simulink model "cruise_ctrl_RL"  (R2021a)
settings: Solver=FixedStepAuto  StartTime=0.0  StopTime=Tf  FixedStep=0.1  RelTol=1e-3
values from neighbouring files (symbols this model uses):
  A = 2.4    [init_cc.m]
  alpha = [40, 25, 16, 12, 10]    [init_cc.m]    (also in main_script_random.m = 0.5)
  beta = 0.4    [init_cc.m]
  Cd = 0.32    [init_cc.m]
  Cr = 0.01    [init_cc.m]
  g = 9.8    [init_cc.m]
  gear = 4    [init_cc.m]
  m = 1000    [init_cc.m]
  rho = 1.3    [init_cc.m]
  Tm = 190    [init_cc.m]
  Ts = 1    [model_myscript.m]    (also in model_myscript_3layer.m)
  wm = 420    [init_cc.m]
undefined symbols (not defined in the file or in its folder): DiscIntNeverNeededParam, phi_cc
libraries: simulink x3, rllib x1
settings Model: Creator=nikhil  LastModifiedBy=nikhil
settings SolverCC: AlgebraicLoopSolver=TrustRegion
settings DataIOCC: ReturnWorkspaceOutputs=off
settings DebuggingCC: SFMachineParentedDataDiag=warning  ArithmeticOperatorsInVariantConditions=warning
settings SFSimCC: SimUseLocalCustomCode=off  CustomCodeUndefinedFunction=UseInterfaceOnly
settings RTWCC: RTWUseLocalCustomCode=off
settings CodeAppCC: StateflowObjectComments=on

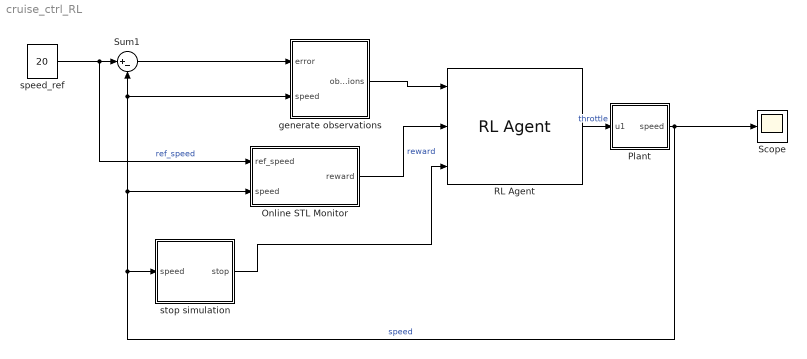
== system cruise_ctrl_RL ==
  Online STL Monitor : Subsystem
  Plant : Subsystem
  RL Agent : rllib/RL Agent  Agent=agent  ExternalActionAsInput=off  ProvideCumRwd=off  TreatAsDirectFeedthrough=on
  Scope : Scope
  Sum1 : Sum  Inputs=|+-  SaturateOnIntegerOverflow=on
  generate observations : Subsystem
  speed_ref : Constant  Value=20
  stop simulation : Subsystem
  wires:
  Plant/1(speed) -> Scope/1, stop simulation/1(speed), Online STL Monitor/2(speed), generate observations/2(speed), Sum1/2  "speed"
  RL Agent/1 -> Plant/1(u1)  "throttle"
  speed_ref/1 -> Online STL Monitor/1(ref_speed), Sum1/1  "ref_speed"
  stop simulation/1(stop) -> RL Agent/3
  generate observations/1(observations) -> RL Agent/1
  Sum1/1 -> generate observations/1(error)
  Online STL Monitor/1(reward) -> RL Agent/2  "reward"

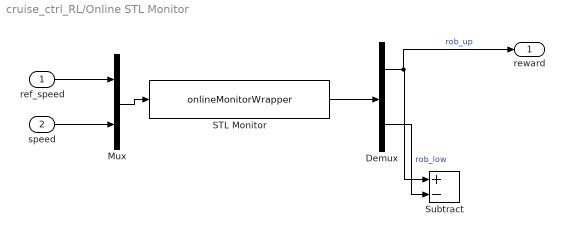
== system cruise_ctrl_RL/Online STL Monitor ==
  ref_speed : Inport
  speed : Inport  Port=2
  Demux : Demux  Outputs=2
  Mux : Mux  Inputs=2
  STL Monitor : S-Function  FunctionName=onlineMonitorWrapper  Parameters=SignalNames, STLString, MaxRob,RefreshRate  SFunctionDeploymentMode=off  EnableBusSupport=off  mask(STL Monitor){SignalNames='ref_speed,speed', STLString=phi_cc, MaxRob=100, RefreshRate=0.1}
      mask prompts: SignalNames "Signal names"; STLString "String For STL formula"; MaxRob "Maximum robustness"; RefreshRate "Refresh Rate"
      mask help:
      | Monitor an STL Formula on input signal. Takes two parameters: a string with
      | comma separated identifiers for the input signals, (ex: 'x1,x2,y'), and a
      | string for the formula (ex: 'alw_[0, 50] (x1[t]>0 => y[t] >0)'). Outputs a
      | two dimensional signal bounding the satisfaction of the formula.
      mask Display: fprintf('%s', STLString)
  Subtract : Sum  Inputs=+-
  reward : Outport
  wires:
  Mux/1 -> STL Monitor/1
  STL Monitor/1 -> Demux/1
  Demux/2 -> Subtract/2  "rob_low"
  Demux/1 -> reward/1, Subtract/1  "rob_up"
  speed/1 -> Mux/2
  ref_speed/1 -> Mux/1

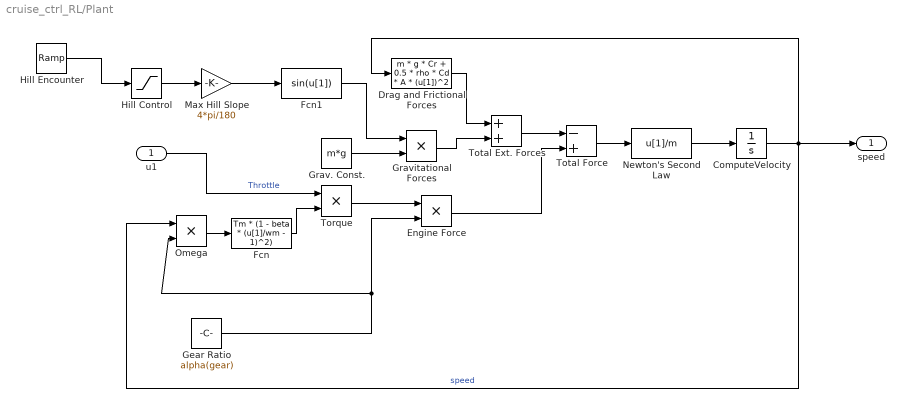
== system cruise_ctrl_RL/Plant ==
  u1 : Inport
  ComputeVelocity : Integrator  InitialCondition=10
  Drag and Frictional Forces : Fcn  Expr=m * g * Cr + 0.5 * rho * Cd * A * (u[1])^2
  Engine Force : Product  Inputs=**
  Fcn : Fcn  Expr=Tm * (1 - beta * (u[1]/wm - 1)^2)
  Fcn1 : Fcn
  Gear Ratio : Constant  Value=alpha(gear)
  Grav. Const. : Constant  Value=m*g
  Gravitational Forces : Product  RndMeth=Zero
  Hill Control : Saturate  UpperLimit=1  LowerLimit=0
  Hill Encounter : simulink/Sources/Ramp  slope=1  start=60  InitialOutput=0
  Max Hill Slope : Gain  Gain=4*pi/180
  Newton's Second Law : Fcn  Expr=u[1]/m
  Omega : Product  RndMeth=Zero
  Torque : Product  RndMeth=Zero
  Total Ext. Forces : Sum
  Total Force : Sum  Inputs=-+
  speed : Outport
  wires:
  Max Hill Slope/1 -> Fcn1/1
  Engine Force/1 -> Total Force/2
  Total Force/1 -> Newton's Second Law/1
  Gravitational Forces/1 -> Total Ext. Forces/2
  Gear Ratio/1 -> Engine Force/2, Omega/2
  Drag and Frictional Forces/1 -> Total Ext. Forces/1
  Total Ext. Forces/1 -> Total Force/1
  Fcn/1 -> Torque/2
  Hill Control/1 -> Max Hill Slope/1
  Hill Encounter/1 -> Hill Control/1
  Fcn1/1 -> Gravitational Forces/1
  Grav. Const./1 -> Gravitational Forces/2
  u1/1 -> Torque/1  "Throttle"
  Torque/1 -> Engine Force/1
  Newton's Second Law/1 -> ComputeVelocity/1
  Omega/1 -> Fcn/1
  ComputeVelocity/1 -> speed/1, Drag and Frictional Forces/1, Omega/1  "speed"

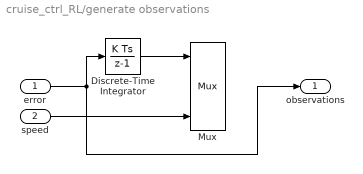
== system cruise_ctrl_RL/generate observations ==
  error : Inport
  speed : Inport  Port=2
  Discrete-Time Integrator : DiscreteIntegrator  SampleTime=Ts  ICPrevOutput=DiscIntNeverNeededParam  ICPrevScaledInput=DiscIntNeverNeededParam
  Mux : Mux  Inputs=3
  observations : Outport  VectorParamsAs1DForOutWhenUnconnected=off
  wires:
  speed/1 -> Mux/3
  Discrete-Time Integrator/1 -> Mux/1
  error/1 -> observations/1, Discrete-Time Integrator/1

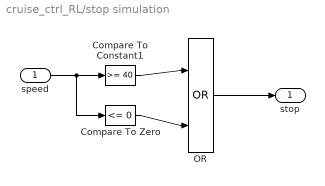
== system cruise_ctrl_RL/stop simulation ==
  speed : Inport
  Compare To Constant1 : simulink/Logic and Bit Operations/Compare To Constant  relop=>=  const=40  OutDataTypeStr=boolean
  Compare To Zero : simulink/Logic and Bit Operations/Compare To Zero  relop=<=  OutDataTypeStr=boolean
  OR : Logic  Operator=OR  IconShape=distinctive  AllPortsSameDT=off  OutDataTypeStr=boolean
  stop : Outport  VectorParamsAs1DForOutWhenUnconnected=off
  wires:
  speed/1 -> Compare To Zero/1, Compare To Constant1/1
  Compare To Zero/1 -> OR/2
  Compare To Constant1/1 -> OR/1
  OR/1 -> stop/1
